simulink model "es3_sim"  (R2022b)
settings: Solver=VariableStepAuto  StartTime=0.0  StopTime=1000  RelTol=1e-3
undefined symbols (not defined in the file): b, d, g, m, x0
settings Model: Creator=claudio  LastModifiedBy=claudio

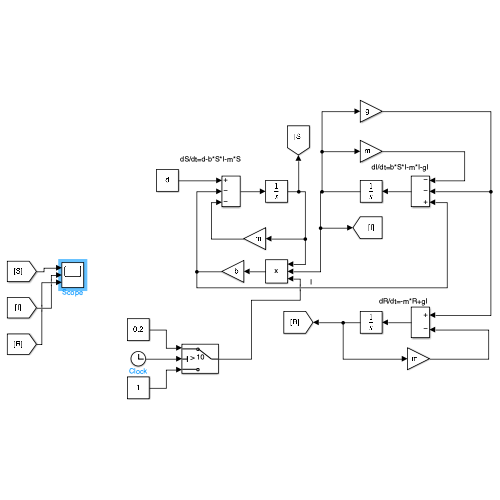
[thumbnail: Simulink's stored preview of the top-level diagram]
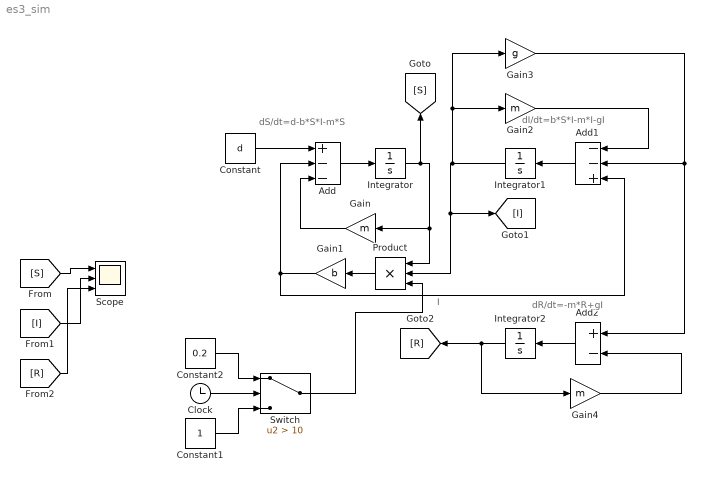
== system es3_sim ==
  note: I
  note: dS/dt=d-b*S*I-m*S
  note: dI/dt=b*S*I-m*I-gI
  note: dR/dt=-m*R+gI
  Add : Sum  Inputs=+--
  Add1 : Sum  Inputs=--+
  Add2 : Sum  Inputs=+-
  Clock : Clock
  Constant : Constant  Value=d
  Constant1 : Constant
  Constant2 : Constant  Value=0.2
  Gain : Gain  Gain=m
  Gain1 : Gain  Gain=b
  Gain2 : Gain  Gain=m
  Gain3 : Gain  Gain=g
  Gain4 : Gain  Gain=m
  Integrator : Integrator  InitialCondition=x0(1)
  Integrator1 : Integrator  InitialCondition=x0(2)
  Integrator2 : Integrator  InitialCondition=x0(3)
  Product : Product  Inputs=3
  Scope : Scope  NumInputPorts=3
  Switch : Switch  Criteria=u2 > Threshold  Threshold=10  SaturateOnIntegerOverflow=off  InputSameDT=off
  wires:
  Add/1 -> Integrator/1
  Constant/1 -> Add/1
  Integrator/1 -> [S], Product/1, Gain/1
  Gain/1 -> Add/3
  Gain1/1 -> Add/2, Add1/3
  Product/1 -> Gain1/1
  Integrator1/1 -> Gain3/1, Gain2/1, [I], Product/2
  Add1/1 -> Integrator1/1
  Gain2/1 -> Add1/1
  Gain3/1 -> Add2/1, Add1/2
  Add2/1 -> Integrator2/1
  Integrator2/1 -> Gain4/1, [R]
  Gain4/1 -> Add2/2
  [S] -> Scope/1
  [I] -> Scope/2
  [R] -> Scope/3
  Clock/1 -> Switch/2
  Constant1/1 -> Switch/3
  Constant2/1 -> Switch/1
  Switch/1 -> Product/3
